simulink model "exo2_Part2_y"  (R2020b)
settings: Solver=VariableStepAuto  StartTime=0.0  StopTime=30  RelTol=1e-3
undefined symbols (not defined in the file or in its folder): fdesignblkfcn, gcbh
libraries: dspfdesign x4, vrlib x1
settings Model: Creator=Hocine
settings DebuggingCC: UnconnectedInputMsg=none  UnconnectedOutputMsg=none  UnconnectedLineMsg=none
settings ModelReferenceCC: EnableRefExpFcnMdlSchedulingChecks=off

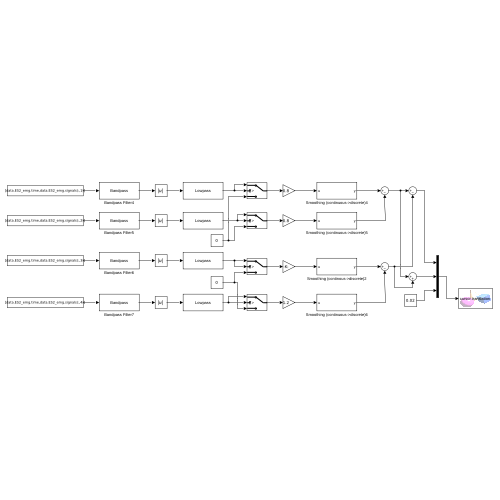
[thumbnail: Simulink's stored preview of the top-level diagram]
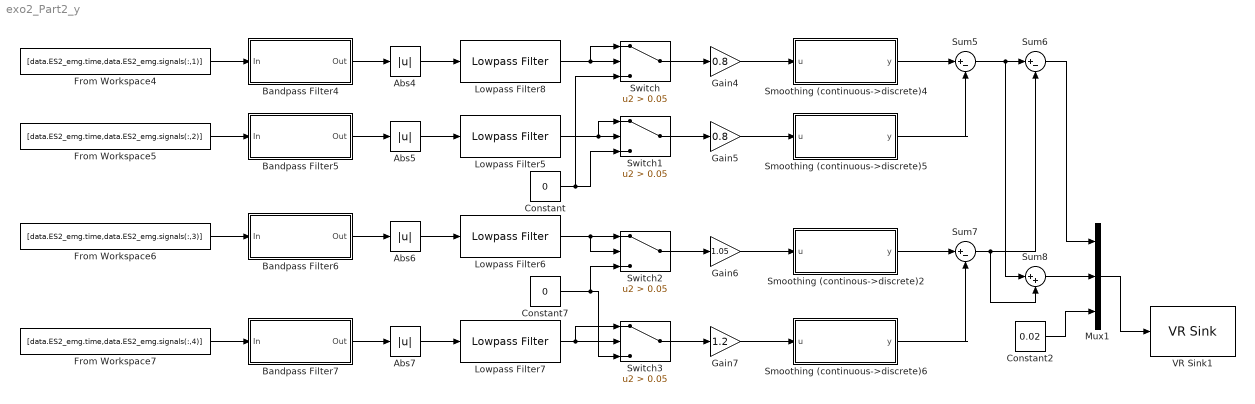
== system exo2_Part2_y ==
  Abs{4..7} (4 alike) : Abs
  Bandpass Filter4 : Subsystem  DialogController=fdesignblkfcn  InitFcn=fdesignblkfcn(gcbh, {'InitFcn'});  mask(Bandpass Filter){}
      mask help: Design a bandpass filter
      settings: CopyFcn=fdesignblkfcn(gcbh, {'CopyFcn'});
      mask Help: helpview(mapfilelocation('dsp'), 'dspbandpassfilter');
      mask Display: disp('Bandpass');
  Bandpass Filter5 : Subsystem  DialogController=fdesignblkfcn  InitFcn=fdesignblkfcn(gcbh, {'InitFcn'});  mask(Bandpass Filter){}
      mask help: Design a bandpass filter
      settings: CopyFcn=fdesignblkfcn(gcbh, {'CopyFcn'});
      mask Help: helpview(mapfilelocation('dsp'), 'dspbandpassfilter');
      mask Display: disp('Bandpass');
  Bandpass Filter6 : Subsystem  DialogController=fdesignblkfcn  InitFcn=fdesignblkfcn(gcbh, {'InitFcn'});  mask(Bandpass Filter){}
      mask help: Design a bandpass filter
      settings: CopyFcn=fdesignblkfcn(gcbh, {'CopyFcn'});
      mask Help: helpview(mapfilelocation('dsp'), 'dspbandpassfilter');
      mask Display: disp('Bandpass');
  Bandpass Filter7 : Subsystem  DialogController=fdesignblkfcn  InitFcn=fdesignblkfcn(gcbh, {'InitFcn'});  mask(Bandpass Filter){}
      mask help: Design a bandpass filter
      settings: CopyFcn=fdesignblkfcn(gcbh, {'CopyFcn'});
      mask Help: helpview(mapfilelocation('dsp'), 'dspbandpassfilter');
      mask Display: disp('Bandpass');
  Constant : Constant  Value=0
  Constant2 : Constant  Value=0.02
  Constant7 : Constant  Value=0
  From Workspace4 : FromWorkspace  VariableName=[data.ES2_emg.time,data.ES2_emg.signals(:,1)]  SampleTime=1/3000
  From Workspace5 : FromWorkspace  VariableName=[data.ES2_emg.time,data.ES2_emg.signals(:,2)]  SampleTime=1/3000
  From Workspace6 : FromWorkspace  VariableName=[data.ES2_emg.time,data.ES2_emg.signals(:,3)]  SampleTime=1/3000
  From Workspace7 : FromWorkspace  VariableName=[data.ES2_emg.time,data.ES2_emg.signals(:,4)]  SampleTime=1/3000
  Gain4 : Gain  Gain=0.8
  Gain5 : Gain  Gain=0.8
  Gain6 : Gain  Gain=1.05
  Gain7 : Gain  Gain=1.2
  Lowpass Filter{5..8} (4 alike) : dspfdesign/Lowpass Filter  InheritSampleRate=off  FilterType=FIR  DesignForMinimumOrder=on  FilterOrder=50  PassbandFrequency=3  StopbandFrequency=6  PassbandRipple=0.1  StopbandAttenuation=80  SampleRate=1000  SimulateUsing=Interpreted execution  roundingMode=Floor  coeffsDataTypeStr=fixdt(1,16)
  Mux1 : Mux  Inputs=3
  Smoothing (continous->discrete)2 : Subsystem  mask(Smoothing (continuous->discrete)){tsSmoothing=0.35, smoothing0=0}
      mask prompts: tsSmoothing "physmod:simscape:couplers:SimscapeNetworkCouplersLib:SmoothingTimeConstants_MP"; smoothing0 "physmod:simscape:couplers:SimscapeNetworkCouplersLib:InitialOutput_MP"
      mask help: physmod:simscape:couplers:SimscapeNetworkCouplersLib:Smoothingcontinuousdiscrete_MD
      mask Help: web([docroot '/physmod/simscape/ref/networkcouplersmoothingcontinuousdiscrete.html'])
      mask DialogControl tsSmoothing Prompt: Smoothing time constant (s)
      mask DialogControl smoothing0 Prompt: Initial output
  Smoothing (continuous->discrete)4 : Subsystem  mask(Smoothing (continuous->discrete)){tsSmoothing=0.35, smoothing0=0}
      mask prompts: tsSmoothing "physmod:simscape:couplers:SimscapeNetworkCouplersLib:SmoothingTimeConstants_MP"; smoothing0 "physmod:simscape:couplers:SimscapeNetworkCouplersLib:InitialOutput_MP"
      mask help: physmod:simscape:couplers:SimscapeNetworkCouplersLib:Smoothingcontinuousdiscrete_MD
      mask Help: web([docroot '/physmod/simscape/ref/networkcouplersmoothingcontinuousdiscrete.html'])
      mask DialogControl tsSmoothing Prompt: Smoothing time constant (s)
      mask DialogControl smoothing0 Prompt: Initial output
  Smoothing (continuous->discrete)5 : Subsystem  mask(Smoothing (continuous->discrete)){tsSmoothing=0.35, smoothing0=0}
      mask prompts: tsSmoothing "physmod:simscape:couplers:SimscapeNetworkCouplersLib:SmoothingTimeConstants_MP"; smoothing0 "physmod:simscape:couplers:SimscapeNetworkCouplersLib:InitialOutput_MP"
      mask help: physmod:simscape:couplers:SimscapeNetworkCouplersLib:Smoothingcontinuousdiscrete_MD
      mask Help: web([docroot '/physmod/simscape/ref/networkcouplersmoothingcontinuousdiscrete.html'])
      mask DialogControl tsSmoothing Prompt: Smoothing time constant (s)
      mask DialogControl smoothing0 Prompt: Initial output
  Smoothing (continuous->discrete)6 : Subsystem  mask(Smoothing (continuous->discrete)){tsSmoothing=0.35, smoothing0=0}
      mask prompts: tsSmoothing "physmod:simscape:couplers:SimscapeNetworkCouplersLib:SmoothingTimeConstants_MP"; smoothing0 "physmod:simscape:couplers:SimscapeNetworkCouplersLib:InitialOutput_MP"
      mask help: physmod:simscape:couplers:SimscapeNetworkCouplersLib:Smoothingcontinuousdiscrete_MD
      mask Help: web([docroot '/physmod/simscape/ref/networkcouplersmoothingcontinuousdiscrete.html'])
      mask DialogControl tsSmoothing Prompt: Smoothing time constant (s)
      mask DialogControl smoothing0 Prompt: Initial output
  Sum5 : Sum  Inputs=|+-
  Sum6 : Sum  Inputs=|+-
  Sum7 : Sum  Inputs=|+-
  Sum8 : Sum  Inputs=|++
  Switch{,1..3} (4 alike) : Switch  Criteria=u2 > Threshold  Threshold=0.05
  VR Sink1 : vrlib/VR Sink  InstantiateOnLoad=on  SampleTime=0.1  ViewEnable=on  RemoteChange=off  RemoteView=off  FieldsWritten=cursor.translation.3.1.1.double  WorldFileName=8_palline_color.wrl  AutoView=off  VideoDimensions=[]  AllowVariableSize=off  FigureProperties=[]
  wires:
  Sum8/1 -> Mux1/2
  Sum6/1 -> Mux1/1
  From Workspace4/1 -> Bandpass Filter4/1(In)
  Gain5/1 -> Smoothing (continuous->discrete)5/1(u)
  Switch/1 -> Gain4/1
  Abs5/1 -> Lowpass Filter5/1
  From Workspace5/1 -> Bandpass Filter5/1(In)
  Abs4/1 -> Lowpass Filter8/1
  Bandpass Filter6/1(Out) -> Abs6/1
  Sum7/1 -> Sum6/2, Sum8/2
  Bandpass Filter5/1(Out) -> Abs5/1
  Abs7/1 -> Lowpass Filter7/1
  Bandpass Filter4/1(Out) -> Abs4/1
  From Workspace6/1 -> Bandpass Filter6/1(In)
  From Workspace7/1 -> Bandpass Filter7/1(In)
  Bandpass Filter7/1(Out) -> Abs7/1
  Sum5/1 -> Sum8/1, Sum6/1
  Gain6/1 -> Smoothing (continous->discrete)2/1(u)
  Switch1/1 -> Gain5/1
  Abs6/1 -> Lowpass Filter6/1
  Lowpass Filter8/1 -> Switch/1, Switch/2
  Lowpass Filter5/1 -> Switch1/1, Switch1/2
  Constant/1 -> Switch/3, Switch1/3
  Lowpass Filter6/1 -> Switch2/1, Switch2/2
  Constant7/1 -> Switch3/3, Switch2/3
  Lowpass Filter7/1 -> Switch3/1, Switch3/2
  Switch2/1 -> Gain6/1
  Switch3/1 -> Gain7/1
  Gain7/1 -> Smoothing (continuous->discrete)6/1(u)
  Gain4/1 -> Smoothing (continuous->discrete)4/1(u)
  Smoothing (continuous->discrete)4/1(y) -> Sum5/1
  Smoothing (continuous->discrete)5/1(y) -> Sum5/2
  Smoothing (continous->discrete)2/1(y) -> Sum7/1
  Smoothing (continuous->discrete)6/1(y) -> Sum7/2
  Constant2/1 -> Mux1/3
  Mux1/1 -> VR Sink1/1

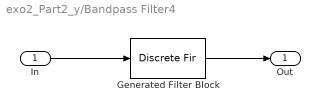
== system exo2_Part2_y/Bandpass Filter4 ==
  In : Inport
  Generated Filter Block : DiscreteFir  Tag=BlockMethodSubSystem  Coefficients=[0.0247784165301624219 0.00982645761122756187 -0.0769563643099292205 -0.00574234407939050277 -0.0280411528162790198 -0.00804608705322145713 -0.0118695570715926946 -0.00997698951682132046 -0.00329006828821561646 -0.0123964456094047496 0.00352600878115868956 -0.0139189700142881862 0.00905023941727299899 -0.0130997642055634047 0.0124656128815528542 -0.00909287544946306772 0.0131317697099942125 -0.00207947540041775744 0.0111769210630364973 0.00659009778413345744 0.0076527361339452345 0.0147232835745344948 0.00427867752511992567 0.0199633122366018496 0.00267711132018834006 0.0203811397583990063 0.00374189409500654642 0.0149169811807582445 0.00742876303379193074 0.00413015922899513752 0.012325804952197969 -0.00967745920215429094 0.0157602502038259491 -0.0236422789640420815 0.0148621759121688127 -0.0338874815186635814 0.00685197471547626009 -0.0377812878977663719 -0.00958300552505605106 -0.0336540649346101367 -0.0340410723239204169 -0.022050280538555421 -0.0639422068094976648 -0.00527010472050308543 -0.0951066582635563262 0.0128546225834286001 -0.122454738580813904 0.02805482821142357 -0.141172435722598549 0.0367254315914400942 0.852170468203799825 0.0367254315914400942 -0.141172435722598549 0.02805482821142357 -0.122454738580813904 0.0128546225834286001 -0.0951066582635563262 -0.00527010472050308543 -0.0639422068094976648 -0.022050280538555421 -0.0340410723239204169 -0.0336540649346101367 -0.00958300552505605106 -0.0377812878977663719 0.00685197471547626009 -0.0338874815186635814 0.0148621759121688127 -0.0236422789640420815 0.0157602502038259491 -0.00967745920215429094 0.012325804952197969 0.00413015922899513752 0.00742876303379193074 0.0149169811807582445 0.00374189409500654642 0.0203811397583990063 0.00267711132018834006 0.0199633122366018496 0.00427867752511992567 0.0147232835745344948 0.0076527361339452345 0.00659009778413345744 0.0111769210630364973 -0.00207947540041775744 0.0131317697099942125 -0.00909287544946306772 0.0124656128815528542 -0.0130997642055634047 0.00905023941727299899 -0.0139189700142881862 0.00352600878115868956 -0.0123964456094047496 -0.00329006828821561646 -0.00997698951682132046 -0.0118695570715926946 -0.00804608705322145713 -0.0280411528162790198 -0.00574234407939050277 -0.0769563643099292205 0.00982645761122756187 0.0247784165301624219]  InputProcessing=Columns as channels (frame based)
  Out : Outport  VectorParamsAs1DForOutWhenUnconnected=off
  wires:
  In/1 -> Generated Filter Block/1
  Generated Filter Block/1 -> Out/1

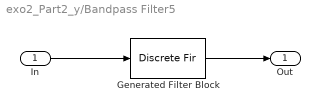
== system exo2_Part2_y/Bandpass Filter5 ==
  In : Inport
  Generated Filter Block : DiscreteFir  Tag=BlockMethodSubSystem  Coefficients=[0.0247784165301624219 0.00982645761122756187 -0.0769563643099292205 -0.00574234407939050277 -0.0280411528162790198 -0.00804608705322145713 -0.0118695570715926946 -0.00997698951682132046 -0.00329006828821561646 -0.0123964456094047496 0.00352600878115868956 -0.0139189700142881862 0.00905023941727299899 -0.0130997642055634047 0.0124656128815528542 -0.00909287544946306772 0.0131317697099942125 -0.00207947540041775744 0.0111769210630364973 0.00659009778413345744 0.0076527361339452345 0.0147232835745344948 0.00427867752511992567 0.0199633122366018496 0.00267711132018834006 0.0203811397583990063 0.00374189409500654642 0.0149169811807582445 0.00742876303379193074 0.00413015922899513752 0.012325804952197969 -0.00967745920215429094 0.0157602502038259491 -0.0236422789640420815 0.0148621759121688127 -0.0338874815186635814 0.00685197471547626009 -0.0377812878977663719 -0.00958300552505605106 -0.0336540649346101367 -0.0340410723239204169 -0.022050280538555421 -0.0639422068094976648 -0.00527010472050308543 -0.0951066582635563262 0.0128546225834286001 -0.122454738580813904 0.02805482821142357 -0.141172435722598549 0.0367254315914400942 0.852170468203799825 0.0367254315914400942 -0.141172435722598549 0.02805482821142357 -0.122454738580813904 0.0128546225834286001 -0.0951066582635563262 -0.00527010472050308543 -0.0639422068094976648 -0.022050280538555421 -0.0340410723239204169 -0.0336540649346101367 -0.00958300552505605106 -0.0377812878977663719 0.00685197471547626009 -0.0338874815186635814 0.0148621759121688127 -0.0236422789640420815 0.0157602502038259491 -0.00967745920215429094 0.012325804952197969 0.00413015922899513752 0.00742876303379193074 0.0149169811807582445 0.00374189409500654642 0.0203811397583990063 0.00267711132018834006 0.0199633122366018496 0.00427867752511992567 0.0147232835745344948 0.0076527361339452345 0.00659009778413345744 0.0111769210630364973 -0.00207947540041775744 0.0131317697099942125 -0.00909287544946306772 0.0124656128815528542 -0.0130997642055634047 0.00905023941727299899 -0.0139189700142881862 0.00352600878115868956 -0.0123964456094047496 -0.00329006828821561646 -0.00997698951682132046 -0.0118695570715926946 -0.00804608705322145713 -0.0280411528162790198 -0.00574234407939050277 -0.0769563643099292205 0.00982645761122756187 0.0247784165301624219]  InputProcessing=Columns as channels (frame based)
  Out : Outport  VectorParamsAs1DForOutWhenUnconnected=off
  wires:
  In/1 -> Generated Filter Block/1
  Generated Filter Block/1 -> Out/1

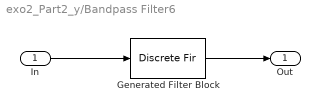
== system exo2_Part2_y/Bandpass Filter6 ==
  In : Inport
  Generated Filter Block : DiscreteFir  Tag=BlockMethodSubSystem  Coefficients=[0.0247784165301624219 0.00982645761122756187 -0.0769563643099292205 -0.00574234407939050277 -0.0280411528162790198 -0.00804608705322145713 -0.0118695570715926946 -0.00997698951682132046 -0.00329006828821561646 -0.0123964456094047496 0.00352600878115868956 -0.0139189700142881862 0.00905023941727299899 -0.0130997642055634047 0.0124656128815528542 -0.00909287544946306772 0.0131317697099942125 -0.00207947540041775744 0.0111769210630364973 0.00659009778413345744 0.0076527361339452345 0.0147232835745344948 0.00427867752511992567 0.0199633122366018496 0.00267711132018834006 0.0203811397583990063 0.00374189409500654642 0.0149169811807582445 0.00742876303379193074 0.00413015922899513752 0.012325804952197969 -0.00967745920215429094 0.0157602502038259491 -0.0236422789640420815 0.0148621759121688127 -0.0338874815186635814 0.00685197471547626009 -0.0377812878977663719 -0.00958300552505605106 -0.0336540649346101367 -0.0340410723239204169 -0.022050280538555421 -0.0639422068094976648 -0.00527010472050308543 -0.0951066582635563262 0.0128546225834286001 -0.122454738580813904 0.02805482821142357 -0.141172435722598549 0.0367254315914400942 0.852170468203799825 0.0367254315914400942 -0.141172435722598549 0.02805482821142357 -0.122454738580813904 0.0128546225834286001 -0.0951066582635563262 -0.00527010472050308543 -0.0639422068094976648 -0.022050280538555421 -0.0340410723239204169 -0.0336540649346101367 -0.00958300552505605106 -0.0377812878977663719 0.00685197471547626009 -0.0338874815186635814 0.0148621759121688127 -0.0236422789640420815 0.0157602502038259491 -0.00967745920215429094 0.012325804952197969 0.00413015922899513752 0.00742876303379193074 0.0149169811807582445 0.00374189409500654642 0.0203811397583990063 0.00267711132018834006 0.0199633122366018496 0.00427867752511992567 0.0147232835745344948 0.0076527361339452345 0.00659009778413345744 0.0111769210630364973 -0.00207947540041775744 0.0131317697099942125 -0.00909287544946306772 0.0124656128815528542 -0.0130997642055634047 0.00905023941727299899 -0.0139189700142881862 0.00352600878115868956 -0.0123964456094047496 -0.00329006828821561646 -0.00997698951682132046 -0.0118695570715926946 -0.00804608705322145713 -0.0280411528162790198 -0.00574234407939050277 -0.0769563643099292205 0.00982645761122756187 0.0247784165301624219]  InputProcessing=Columns as channels (frame based)
  Out : Outport  VectorParamsAs1DForOutWhenUnconnected=off
  wires:
  In/1 -> Generated Filter Block/1
  Generated Filter Block/1 -> Out/1

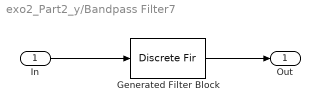
== system exo2_Part2_y/Bandpass Filter7 ==
  In : Inport
  Generated Filter Block : DiscreteFir  Tag=BlockMethodSubSystem  Coefficients=[0.0247784165301624219 0.00982645761122756187 -0.0769563643099292205 -0.00574234407939050277 -0.0280411528162790198 -0.00804608705322145713 -0.0118695570715926946 -0.00997698951682132046 -0.00329006828821561646 -0.0123964456094047496 0.00352600878115868956 -0.0139189700142881862 0.00905023941727299899 -0.0130997642055634047 0.0124656128815528542 -0.00909287544946306772 0.0131317697099942125 -0.00207947540041775744 0.0111769210630364973 0.00659009778413345744 0.0076527361339452345 0.0147232835745344948 0.00427867752511992567 0.0199633122366018496 0.00267711132018834006 0.0203811397583990063 0.00374189409500654642 0.0149169811807582445 0.00742876303379193074 0.00413015922899513752 0.012325804952197969 -0.00967745920215429094 0.0157602502038259491 -0.0236422789640420815 0.0148621759121688127 -0.0338874815186635814 0.00685197471547626009 -0.0377812878977663719 -0.00958300552505605106 -0.0336540649346101367 -0.0340410723239204169 -0.022050280538555421 -0.0639422068094976648 -0.00527010472050308543 -0.0951066582635563262 0.0128546225834286001 -0.122454738580813904 0.02805482821142357 -0.141172435722598549 0.0367254315914400942 0.852170468203799825 0.0367254315914400942 -0.141172435722598549 0.02805482821142357 -0.122454738580813904 0.0128546225834286001 -0.0951066582635563262 -0.00527010472050308543 -0.0639422068094976648 -0.022050280538555421 -0.0340410723239204169 -0.0336540649346101367 -0.00958300552505605106 -0.0377812878977663719 0.00685197471547626009 -0.0338874815186635814 0.0148621759121688127 -0.0236422789640420815 0.0157602502038259491 -0.00967745920215429094 0.012325804952197969 0.00413015922899513752 0.00742876303379193074 0.0149169811807582445 0.00374189409500654642 0.0203811397583990063 0.00267711132018834006 0.0199633122366018496 0.00427867752511992567 0.0147232835745344948 0.0076527361339452345 0.00659009778413345744 0.0111769210630364973 -0.00207947540041775744 0.0131317697099942125 -0.00909287544946306772 0.0124656128815528542 -0.0130997642055634047 0.00905023941727299899 -0.0139189700142881862 0.00352600878115868956 -0.0123964456094047496 -0.00329006828821561646 -0.00997698951682132046 -0.0118695570715926946 -0.00804608705322145713 -0.0280411528162790198 -0.00574234407939050277 -0.0769563643099292205 0.00982645761122756187 0.0247784165301624219]  InputProcessing=Columns as channels (frame based)
  Out : Outport  VectorParamsAs1DForOutWhenUnconnected=off
  wires:
  In/1 -> Generated Filter Block/1
  Generated Filter Block/1 -> Out/1

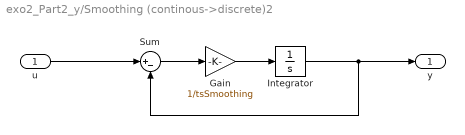
== system exo2_Part2_y/Smoothing (continous->discrete)2 ==
  u : Inport
  Gain : Gain  Gain=1/tsSmoothing
  Integrator : Integrator  InitialCondition=smoothing0
  Sum : Sum  Inputs=|+-
  y : Outport
  wires:
  u/1 -> Sum/1
  Integrator/1 -> Sum/2, y/1
  Gain/1 -> Integrator/1
  Sum/1 -> Gain/1

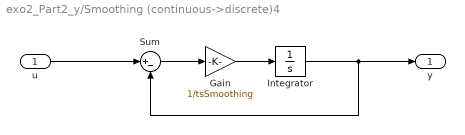
== system exo2_Part2_y/Smoothing (continuous->discrete)4 ==
  u : Inport
  Gain : Gain  Gain=1/tsSmoothing
  Integrator : Integrator  InitialCondition=smoothing0
  Sum : Sum  Inputs=|+-
  y : Outport
  wires:
  u/1 -> Sum/1
  Integrator/1 -> Sum/2, y/1
  Gain/1 -> Integrator/1
  Sum/1 -> Gain/1

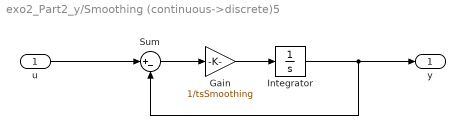
== system exo2_Part2_y/Smoothing (continuous->discrete)5 ==
  u : Inport
  Gain : Gain  Gain=1/tsSmoothing
  Integrator : Integrator  InitialCondition=smoothing0
  Sum : Sum  Inputs=|+-
  y : Outport
  wires:
  u/1 -> Sum/1
  Integrator/1 -> Sum/2, y/1
  Gain/1 -> Integrator/1
  Sum/1 -> Gain/1

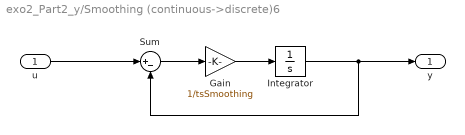
== system exo2_Part2_y/Smoothing (continuous->discrete)6 ==
  u : Inport
  Gain : Gain  Gain=1/tsSmoothing
  Integrator : Integrator  InitialCondition=smoothing0
  Sum : Sum  Inputs=|+-
  y : Outport
  wires:
  u/1 -> Sum/1
  Integrator/1 -> Sum/2, y/1
  Gain/1 -> Integrator/1
  Sum/1 -> Gain/1
